simulink model "SensorFusion_Controller_Model"  (R2025a)
settings: Solver=VariableStepAuto  StartTime=0.0  StopTime=inf  FixedStep=1  RelTol=1e-3
undefined symbols (not defined in the file): DiscIntNeverNeededParam
libraries: simulink x17
(part 3 of 4)

== matlab function SensorFusion_Controller_Model/Sensor Fusion/Radar Sensor 1 ==
  data: dist input; elevation_live output; secondsCounter input; dayCounter input; water_lvl_live output; elevation_daily output
function [elevation_live, water_lvl_live, elevation_daily] = riverElevationSensor(dist, secondsCounter, dayCounter)

% INPUTS:
% dist - radar-measured distance from sensor to water surface (m) comes from the dashboard slider input
% secondsCounter - current second within the day (0 to 86399), from timer
% dayCounter- how many full days have passed, from timer
%
% OUTPUTS (LIVE that updates every timestep, use these for dashboard):
% elevation_live - current smoothed river water elevation in metres
% water_lvl_live - current water level status string (live, for dashboard)
%
% OUTPUTS (DAILY AVERAGE - updates once per day rollover, use for logger):
% elevation_daily - average river elevation across the entire previous day (m) computed as running sum 
% over 86400 seconds
%
% HOW IT WORKS:
% the sensor converts radar distance to river elevation using a fixed reference elevation (ref_elev).
% a smoothing factor gradually moves the elevation toward the target rather than jumping instantly,
% simulating real sensor lag. Every 86400 seconds (1 day), the current live values are saved as
% the daily snapshot before the timer resets.

ref_elev = 5.0; % height of sensor mount above riverbed (metres)
% water elevation = ref_elev - dist
MIN_ELEV = 0.0; % river physically cannot be below 0m
MAX_ELEV = 4.0; % maximum valid river level as defined by project spec

persistent prevSec prevDay elevation elevation_daily_store daily_sum daily_count

% initialise persistent variables
if isempty(prevSec), prevSec = 0; end
if isempty(prevDay), prevDay = 0; end
if isempty(elevation), elevation = ref_elev - dist; end
if isempty(elevation_daily_store), elevation_daily_store = 0; end
if isempty(daily_sum), daily_sum = 0; end
if isempty(daily_count), daily_count = 0; end

% time delta calculation
deltaT = secondsCounter - prevSec;
if deltaT <= 0
    deltaT = 1; % guard against zero or negative delta on reset tick
end

% target_elev is where the reading should be based on current dist input
target_elev = ref_elev - dist;

% clamp the target to valid physical range to prevents the slider going out of range
target_elev = max(MIN_ELEV, min(MAX_ELEV, target_elev));

% gradually move elevation toward target (smoothing factor = 100)
% a higher denominator = slower/smoother response to input changes
rate = (target_elev - elevation) / 100;
elevation = elevation + rate * deltaT;
elevation = max(MIN_ELEV, min(MAX_ELEV, elevation));

% Water level classification (based on live elevation) Thresholds (metres):
% elevation > 2.05 = Normal
% 1.70 < elevation <= 2.05 = Alert
% elevation <= 1.70 = Critical
if elevation > 2.05
    water_lvl_str = "Normal";
elseif elevation > 1.70
    water_lvl_str = "Alert";
else
    water_lvl_str = "Critical";
end

% add current elevation to running sum for daily average calculation
% Simulink calls this function every timestep so daily_sum accumulates all readings across the day,
% daily_count tracks how many readings taken
daily_sum   = daily_sum + elevation;
daily_count = daily_count + 1;

% daily average when the day counter increments
% when dayCounter changes, it means 86400s have passed and the timer reset for new day
if double(dayCounter) ~= double(prevDay)
    if daily_count > 0
        elevation_daily_store = daily_sum / daily_count; % true daily average
    end
    daily_sum   = 0; % reset accumulator for new day
    daily_count = 0; % reset sample counter for new day
    prevDay = double(dayCounter);
end

% update state for next timestep
prevSec = secondsCounter;

% assign outputs
% live outputs to the dashboard signals
elevation_live = elevation;
water_lvl_live = water_lvl_str;

% daily average output to the dailyLogger block
elevation_daily = elevation_daily_store;

end

== matlab function SensorFusion_Controller_Model/Sensor Fusion/MATLAB Function5 ==
  data: r1 input; elevation_fused_live output; r2 input; r3 input; fault_flags output; elevation_fused_daily output; dayCounter input
function [elevation_fused_live, fault_flags, elevation_fused_daily] = fuseRiverElevationSensors(r1, r2, r3, dayCounter)

% INPUTS:
% r1, r2, r3 - live elevation outputs from the 3 river sensor chains (m)
% dayCounter - how many full days have passed, from timer
%
% OUTPUTS (LIVE - updates every timestep, use for dashboard):
% elevation_fused_live - single best-estimate river elevation in metres
% fault_flags - [f1 f2 f3] boolean array, 1 = that sensor is flagged faulty
%
% OUTPUTS (DAILY AVERAGE - updates once per day rollover, use for logger):
% elevation_fused_daily - average fused river elevation across the entire day (m)
% computed as running sum / sample count over 86400 seconds
%
% HOW IT WORKS:
% 1. compute the mean of all 3 sensor readings
% 2. flag any sensor that deviates more than tolerance % from the mean as faulty
% 3. use only the non-faulty sensors to compute the fused value:
% - 3 valid = median
% - 2 valid = mean of the two
% - 1 valid = use that sensor directly
% - 0 valid = fallback to mean of all 3
% 4. hard clamp the output to [MIN_ELEV, MAX_ELEV] regardless of result
% to ensure no out-of-range value ever leaves this block
% 5. accumulate fused live value into running sum every timestep
% on dayCounter increment, compute daily average and reset accumulators

MIN_ELEV = 0.0;
MAX_ELEV = 4.0;
REF_HEIGHT = 5.0;

% fault detection tolerance
tol = 0.05; % sensor flagged if it deviates >5% from mean

% persistent variables for daily average tracking
persistent prevDay daily_sum daily_count fused_daily_store

% initialise persistent variables
if isempty(prevDay),          prevDay = 0;           end
if isempty(daily_sum),        daily_sum = 0;         end
if isempty(daily_count),      daily_count = 0;       end
if isempty(fused_daily_store),fused_daily_store = 0; end

% collect readings and calculate mean
vals = [r1, r2, r3];
mean_val = mean(vals);

% fault detection via comparing to tol % mean value
% use max(mean_val, 0.01) to avoid division by zero when mean is ~0
fault_flags = abs(vals - mean_val) > tol * max(mean_val, 0.01);

% fuse using only valid (non-faulty) sensors
valid_vals = vals(~fault_flags);
if isempty(valid_vals) % all 3 sensors flagged so fall back to best mean of all
    elevation_fused_live = mean_val;
elseif isscalar(valid_vals) % only 1 sensor valid, use it directly
    elevation_fused_live = valid_vals(1);
elseif numel(valid_vals) == 2 % 2 sensors valid, average them
    elevation_fused_live = mean(valid_vals);
else % all 3 sensors valid, use median
    elevation_fused_live = median(valid_vals);
end

% convert fused overhead distance to actual river level/depth
overhead_fused = elevation_fused_live;
elevation_fused_live = REF_HEIGHT - overhead_fused;

% output clamp
elevation_fused_live = max(MIN_ELEV, min(MAX_ELEV, elevation_fused_live));

% add fused value to running sum every timestep
% all readings across the day, daily_count tracks how many readings taken
daily_sum   = daily_sum + elevation_fused_live;
daily_count = daily_count + 1;

% daily average when dayCounter increments
if double(dayCounter) ~= double(prevDay)
    if daily_count > 0
        fused_daily_store = daily_sum / daily_count; % basically moving average
    end
    daily_sum   = 0; % reset accumulator for new day
    daily_count = 0; % reset sample counter for new day
    prevDay     = double(dayCounter);
end

% daily average output to dailyLogger block
elevation_fused_daily = fused_daily_store;

end

== matlab function SensorFusion_Controller_Model/Sensor Fusion/Soil Moisture Probe2 ==
  data: moisture_live output; moisture_type_live output; voltage_live output; sliderInput input; secondsCounter input; dayCounter input; moisture_daily output
function [moisture_live, moisture_type_live, voltage_live, moisture_daily] = soilMoistureProbe(sliderInput, ...
    secondsCounter, dayCounter)

% INPUTS:
% sliderInput - rainfall rate in mm/s from the dashboard slider
% secondsCounter - current second within the day (0 to 86399), from timer
% dayCounter - how many full days have passed, from timer
%
% OUTPUTS (LIVE which updates every timestep, use for dashboard):
% moisture_live - current soil moisture percentage (0 to 100%)
% moisture_type_live - current moisture category string (live)
% voltage_live - current sensor voltage output (live)
%
% OUTPUTS (DAILY - updates once per day rollover, use for logger):
% moisture_daily - end of day soil moisture % captured from previous tick
% scaled so max slider input (0.0012 mm/s) = 100% rounded to nearest whole 
% percentage
%
% HOW IT WORKS:
% Rainfall infiltrates into soil at a given efficiency rate, increasing the volumetric water content (VWC). 
% Evapotranspiration (ET) constantly draws moisture out. The resulting VWC is clamped to 0-100% and mapped
% to a moisture category and analog voltage every 86400 seconds the end-of-day values are snapshotted for 
% the logger
% on dayCounter increment, the daily value is captured from prev_moisture (previous tick's value)
% before resetting VWC to 0 for the new day, same pattern as tipping bucket.
% gain of 4.25 is applied so that max slider input (0.0012 mm/s) maps to 100%
% raw calculation gives 23.52% at max input, scale factor = 100/23.52 = 4.25

% constants
infil_eff = 0.7; % infiltration efficiency (70% of rain enters soil)
d = 300; % effective soil depth (mm)
ET_day = 2; % evapotranspiration loss per day (mm/day)
ET_rate = ET_day / 86400; % ET converted to per-second rate (mm/s)
gain = 4.25; % scale factor so max slider input = 100% (100/23.52 = 4.25)

persistent VWC prevSec prevDay moisture_daily_store prev_moisture

% initialise values
if isempty(VWC), VWC = 0; end
if isempty(prevSec), prevSec = 0; end
if isempty(prevDay), prevDay = 0; end
if isempty(moisture_daily_store), moisture_daily_store = 0; end
if isempty(prev_moisture), prev_moisture = 0; end

% time delta
deltaT = secondsCounter - prevSec;
if deltaT <= 0
    deltaT = 1;
end

% calculate how much rain falls and infiltrates in this timestep
rain_mm  = sliderInput * deltaT; % total rainfall in this timestep (mm)
infil_mm = infil_eff * rain_mm; % portion that actually enters the soil
rain_frac = infil_mm / d; % expressed as fraction of total soil depth

% calculate evapotranspiration loss in this timestep
ET_mm = ET_rate * deltaT; % moisture lost to ET this timestep (mm)
ET_frac = ET_mm / d; % expressed as fraction of total soil depth

% update cumulative volumetric water content in fraction
VWC = VWC + rain_frac - ET_frac;

% convert to raw percentage first (unscaled) for VWC writeback
moisture_pct_raw = VWC * 100;

% apply gain so max slider input = 100%, round and clamp
moisture_pct = round(moisture_pct_raw * gain);
moisture_pct = max(0, min(100, moisture_pct));

% write back using raw unscaled value so VWC accumulates correctly
% do NOT use moisture_pct here as it includes gain which would shrink VWC
VWC = moisture_pct_raw / 100;
VWC = max(0, VWC); % ensure VWC never goes negative

% moisture category classification
% 0  to < 25  = Dry
% 25 to < 50  = Moderate
% 50 to < 75  = Wet
% 75 to 100   = Saturated
if moisture_pct < 25
    moisture_type = "Dry";
elseif moisture_pct < 50
    moisture_type = "Moderate";
elseif moisture_pct < 75
    moisture_type = "Wet";
else
    moisture_type = "Saturated";
end

% voltage output
% 0% moisture = 0.5V
% 100% moisture = 1.5V
voltage = 0.5 + (moisture_pct / 100);

% daily value when the day counter increments
% prev_moisture holds value from previous tick before reset fires
% so we capture true end-of-day value, not post-reset zero
if double(dayCounter) ~= double(prevDay)
    moisture_daily_store = prev_moisture; % capture previous tick's value
    VWC = 0; % reset soil moisture for new day
    prevDay = double(dayCounter);
end

% update state for next timestep
prevSec = secondsCounter;
prev_moisture = moisture_pct; % store current value for next tick's capture

% assign outputs
% live outputs to the dashboard signals
moisture_live = moisture_pct;
moisture_type_live = moisture_type;
voltage_live = voltage;

% daily output to the dailyLogger block
moisture_daily = moisture_daily_store;

end

== matlab function SensorFusion_Controller_Model/Sensor Fusion/Tipping Bucket 1 ==
  data: sliderInput input; rainfall_live output; rainfall_daily output; secondsCounter input; dayCounter input; totalTipsDaily output
function [rainfall_live, rainfall_daily, totalTipsDaily] = tippingBucket1(sliderInput, secondsCounter, dayCounter)

% INPUTS:
% sliderInput - rainfall rate in mm/s from the dashboard slider
% secondsCounter - current second within the day (0 to 86399), from timer
% dayCounter - how many full days have passed, from timer
%
% OUTPUTS (LIVE - updates every timestep, use for dashboard):
% rainfall_live - running rainfall total today in mm
%
% OUTPUTS (DAILY TOTAL - updates once per day rollover, use for logger):
% rainfall_daily - total rainfall for the completed previous day (mm)
% totalTipsDaily  - total tips recorded for the completed previous day
%
% HOW IT WORKS:
% Rain accumulates in a virtual 0.2mm/tip bucket. Every time accumulated water reaches 0.2mm the bucket
% tips, incrementing the tip counter and subtracting 0.2mm from the accumulator.
% Total rainfall = tips * 0.2mm.
% On dayCounter increment, the daily total is captured from the PREVIOUS tick's value
% via prev_rainfall and prev_tips, before resetting counters for the new day.

TIP_VOL = 0.2; % each tip represents 0.2mm of rainfall

persistent acc tips prevSec prevDay rainfall_daily_store totalTips_store prev_rainfall prev_tips

if isempty(acc), acc = 0; end
if isempty(tips), tips = 0; end
if isempty(prevSec), prevSec = 0; end
if isempty(prevDay), prevDay = 0; end
if isempty(rainfall_daily_store), rainfall_daily_store = 0; end
if isempty(totalTips_store), totalTips_store = 0; end
if isempty(prev_rainfall), prev_rainfall = 0; end
if isempty(prev_tips), prev_tips = 0; end

deltaT = secondsCounter - prevSec;
if deltaT <= 0
    deltaT = 1; % guard against zero or negative delta on reset tick
end

% accumulate rainfall and count tips
acc = acc + sliderInput * deltaT;
while acc >= TIP_VOL
    tips = tips + 1; % one tip recorded
    acc  = acc - TIP_VOL; % remove one tip's worth from accumulator
end

% daily rollover to capture total then reset all counters for new day
if double(dayCounter) ~= double(prevDay)
    rainfall_daily_store = prev_rainfall; % capture today's total
    totalTips_store = prev_tips; % capture today's total tip count
    tips = 0; % reset tip counter for new day
    acc = 0; % reset accumulator for new day
    prevDay = double(dayCounter);
end

% update state for next timestep
prevSec = secondsCounter;
prev_rainfall = tips * TIP_VOL; % store current value for next tick's capture
prev_tips = tips; % store current tips for next tick's capture

% assign outputs
rainfall_live  = tips * TIP_VOL; % live running total for dashboard
rainfall_daily = rainfall_daily_store; % daily total for logger
totalTipsDaily = totalTips_store; % daily total tips for display

end

== matlab function SensorFusion_Controller_Model/Sensor Fusion/MATLAB Function6 ==
  data: noisy_input input; x_est output
function x_est = kalmanFilter(noisy_input)

persistent x P
if isempty(x), x = noisy_input; end
if isempty(P), P = 1; end


Q = 1e-10;   % process noise covariance
R = 1e-9;   % measurement noise covariance
% filter will trust measurement more since Q > R

% prediction
x_pred = x;
P_pred = P + Q;

% update
K = P_pred / (P_pred + R);
x = x_pred + K*(noisy_input - x_pred);
P = (1 - K)*P_pred;

x_est = max(0, x);

== matlab function SensorFusion_Controller_Model/Sensor Fusion/MATLAB Function7 ==
  data: noisy_input input; x_est output
function x_est = kalmanFilter(noisy_input)

persistent x P
if isempty(x), x = noisy_input; end
if isempty(P), P = 1; end


Q = 1e-10;   % process noise covariance
R = 1e-9;   % measurement noise covariance
% filter will trust measurement more since Q > R

% prediction
x_pred = x;
P_pred = P + Q;

% update
K = P_pred / (P_pred + R);
x = x_pred + K*(noisy_input - x_pred);
P = (1 - K)*P_pred;

x_est = max(0, x);

== matlab function SensorFusion_Controller_Model/Sensor Fusion/MATLAB Function8 ==
  data: r1 input; rainfall_fused_live output; r2 input; r3 input; fault_flags output; rainfall_fused_daily output; dayCounter input
function [rainfall_fused_live, fault_flags, rainfall_fused_daily] = fuseTippingBucketSensors(r1, r2, r3, dayCounter)
% INPUTS:
% r1, r2, r3 - rainfall_live outputs from the 3 tipping bucket chains (mm)
% dayCounter - how many full days have passed, from timer
%
% OUTPUTS (LIVE - updates every timestep, use for dashboard):
% rainfall_fused_live - single best-estimate running rainfall total in mm
% fault_flags - [f1 f2 f3] boolean array, 1 = that sensor is flagged faulty
%
% OUTPUTS (DAILY TOTAL - updates once per day rollover, use for logger):
% rainfall_fused_daily - total fused rainfall for the completed day (mm)
% captured from the previous tick before tippingBucket resets to 0
%
% HOW IT WORKS:
% same structure as the other fusion blocks with 10% tolerance only unlike soil moisture and river
% elevation and the daily value is a total
% prev_fused stores the fused value from the previous tick so that when
% dayCounter increments on the same tick that sensors reset to 0, we
% capture the true end-of-day total rather than the post-reset zero

% limits
MIN_RAIN = 0.0;
MAX_RAIN = Inf;

% fault detection tolerance
tol = 0.10;
abs_floor = 0.4; % 0.4mm absolute floor to prevents false fault at near-zero

% persistent variables for daily total tracking
persistent prevDay fused_daily_store prev_fused

% initialise persistent variables
if isempty(prevDay), prevDay = 0; end
if isempty(fused_daily_store), fused_daily_store = 0; end
if isempty(prev_fused), prev_fused = 0; end

% calculate mean
vals = [r1, r2, r3];
mean_val = mean(vals);

% fault detection
% sensor is faulty if BOTH the relative AND absolute deviations are large
% using AND logic prevents flagging sensors just because of tiny 0.2mm tip
% differences when all sensors are essentially reading the same thing
rel_dev = abs(vals - mean_val) > tol * max(mean_val, 0.01);
abs_dev = abs(vals - mean_val) > abs_floor;
fault_flags = rel_dev & abs_dev;

% fuse using only valid sensors
valid_vals = vals(~fault_flags);
if isempty(valid_vals)
    rainfall_fused_live = mean_val;
elseif isscalar(valid_vals)
    rainfall_fused_live = valid_vals(1);
elseif numel(valid_vals) == 2
    rainfall_fused_live = mean(valid_vals);
else
    rainfall_fused_live = median(valid_vals);
end

% output clamp
rainfall_fused_live = max(MIN_RAIN, rainfall_fused_live);

% daily total when dayCounter increments
% prev_fused holds the fused value from the tick before the reset
% so we capture the true end-of-day total, not the post-reset 0
if double(dayCounter) ~= double(prevDay)
    fused_daily_store = prev_fused; % use previous tick's value
    prevDay = double(dayCounter);
end

% store current fused value for next tick's capture
prev_fused = rainfall_fused_live;

% daily total output to dailyLogger block
rainfall_fused_daily = fused_daily_store;

end

== matlab function SensorFusion_Controller_Model/Sensor Fusion/Soil Moisture Probe3 ==
  data: moisture_live output; moisture_type_live output; voltage_live output; sliderInput input; secondsCounter input; dayCounter input; moisture_daily output
function [moisture_live, moisture_type_live, voltage_live, moisture_daily] = soilMoistureProbe(sliderInput, ...
    secondsCounter, dayCounter)

% INPUTS:
% sliderInput - rainfall rate in mm/s from the dashboard slider
% secondsCounter - current second within the day (0 to 86399), from timer
% dayCounter - how many full days have passed, from timer
%
% OUTPUTS (LIVE which updates every timestep, use for dashboard):
% moisture_live - current soil moisture percentage (0 to 100%)
% moisture_type_live - current moisture category string (live)
% voltage_live - current sensor voltage output (live)
%
% OUTPUTS (DAILY - updates once per day rollover, use for logger):
% moisture_daily - end of day soil moisture % captured from previous tick
% scaled so max slider input (0.0012 mm/s) = 100% rounded to nearest whole 
% percentage
%
% HOW IT WORKS:
% Rainfall infiltrates into soil at a given efficiency rate, increasing the volumetric water content (VWC). 
% Evapotranspiration (ET) constantly draws moisture out. The resulting VWC is clamped to 0-100% and mapped
% to a moisture category and analog voltage every 86400 seconds the end-of-day values are snapshotted for 
% the logger
% on dayCounter increment, the daily value is captured from prev_moisture (previous tick's value)
% before resetting VWC to 0 for the new day, same pattern as tipping bucket.
% gain of 4.25 is applied so that max slider input (0.0012 mm/s) maps to 100%
% raw calculation gives 23.52% at max input, scale factor = 100/23.52 = 4.25

% constants
infil_eff = 0.7; % infiltration efficiency (70% of rain enters soil)
d = 300; % effective soil depth (mm)
ET_day = 2; % evapotranspiration loss per day (mm/day)
ET_rate = ET_day / 86400; % ET converted to per-second rate (mm/s)
gain = 4.25; % scale factor so max slider input = 100% (100/23.52 = 4.25)

persistent VWC prevSec prevDay moisture_daily_store prev_moisture

% initialise values
if isempty(VWC), VWC = 0; end
if isempty(prevSec), prevSec = 0; end
if isempty(prevDay), prevDay = 0; end
if isempty(moisture_daily_store), moisture_daily_store = 0; end
if isempty(prev_moisture), prev_moisture = 0; end

% time delta
deltaT = secondsCounter - prevSec;
if deltaT <= 0
    deltaT = 1;
end

% calculate how much rain falls and infiltrates in this timestep
rain_mm  = sliderInput * deltaT; % total rainfall in this timestep (mm)
infil_mm = infil_eff * rain_mm; % portion that actually enters the soil
rain_frac = infil_mm / d; % expressed as fraction of total soil depth

% calculate evapotranspiration loss in this timestep
ET_mm = ET_rate * deltaT; % moisture lost to ET this timestep (mm)
ET_frac = ET_mm / d; % expressed as fraction of total soil depth

% update cumulative volumetric water content in fraction
VWC = VWC + rain_frac - ET_frac;

% convert to raw percentage first (unscaled) for VWC writeback
moisture_pct_raw = VWC * 100;

% apply gain so max slider input = 100%, round and clamp
moisture_pct = round(moisture_pct_raw * gain);
moisture_pct = max(0, min(100, moisture_pct));

% write back using raw unscaled value so VWC accumulates correctly
% do NOT use moisture_pct here as it includes gain which would shrink VWC
VWC = moisture_pct_raw / 100;
VWC = max(0, VWC); % ensure VWC never goes negative

% moisture category classification
% 0  to < 25  = Dry
% 25 to < 50  = Moderate
% 50 to < 75  = Wet
% 75 to 100   = Saturated
if moisture_pct < 25
    moisture_type = "Dry";
elseif moisture_pct < 50
    moisture_type = "Moderate";
elseif moisture_pct < 75
    moisture_type = "Wet";
else
    moisture_type = "Saturated";
end

% voltage output
% 0% moisture = 0.5V
% 100% moisture = 1.5V
voltage = 0.5 + (moisture_pct / 100);

% daily value when the day counter increments
% prev_moisture holds value from previous tick before reset fires
% so we capture true end-of-day value, not post-reset zero
if double(dayCounter) ~= double(prevDay)
    moisture_daily_store = prev_moisture; % capture previous tick's value
    VWC = 0; % reset soil moisture for new day
    prevDay = double(dayCounter);
end

% update state for next timestep
prevSec = secondsCounter;
prev_moisture = moisture_pct; % store current value for next tick's capture

% assign outputs
% live outputs to the dashboard signals
moisture_live = moisture_pct;
moisture_type_live = moisture_type;
voltage_live = voltage;

% daily output to the dailyLogger block
moisture_daily = moisture_daily_store;

end

== matlab function SensorFusion_Controller_Model/Sensor Fusion/Soil Moisture Probe1 ==
  data: moisture_live output; moisture_type_live output; voltage_live output; sliderInput input; secondsCounter input; dayCounter input; moisture_daily output
function [moisture_live, moisture_type_live, voltage_live, moisture_daily] = soilMoistureProbe(sliderInput, ...
    secondsCounter, dayCounter)

% INPUTS:
% sliderInput - rainfall rate in mm/s from the dashboard slider
% secondsCounter - current second within the day (0 to 86399), from timer
% dayCounter - how many full days have passed, from timer
%
% OUTPUTS (LIVE which updates every timestep, use for dashboard):
% moisture_live - current soil moisture percentage (0 to 100%)
% moisture_type_live - current moisture category string (live)
% voltage_live - current sensor voltage output (live)
%
% OUTPUTS (DAILY - updates once per day rollover, use for logger):
% moisture_daily - end of day soil moisture % captured from previous tick
% scaled so max slider input (0.0012 mm/s) = 100% rounded to nearest whole 
% percentage
%
% HOW IT WORKS:
% Rainfall infiltrates into soil at a given efficiency rate, increasing the volumetric water content (VWC). 
% Evapotranspiration (ET) constantly draws moisture out. The resulting VWC is clamped to 0-100% and mapped
% to a moisture category and analog voltage every 86400 seconds the end-of-day values are snapshotted for 
% the logger
% on dayCounter increment, the daily value is captured from prev_moisture (previous tick's value)
% before resetting VWC to 0 for the new day, same pattern as tipping bucket.
% gain of 4.25 is applied so that max slider input (0.0012 mm/s) maps to 100%
% raw calculation gives 23.52% at max input, scale factor = 100/23.52 = 4.25

% constants
infil_eff = 0.7; % infiltration efficiency (70% of rain enters soil)
d = 300; % effective soil depth (mm)
ET_day = 2; % evapotranspiration loss per day (mm/day)
ET_rate = ET_day / 86400; % ET converted to per-second rate (mm/s)
gain = 4.25; % scale factor so max slider input = 100% (100/23.52 = 4.25)

persistent VWC prevSec prevDay moisture_daily_store prev_moisture

% initialise values
if isempty(VWC), VWC = 0; end
if isempty(prevSec), prevSec = 0; end
if isempty(prevDay), prevDay = 0; end
if isempty(moisture_daily_store), moisture_daily_store = 0; end
if isempty(prev_moisture), prev_moisture = 0; end

% time delta
deltaT = secondsCounter - prevSec;
if deltaT <= 0
    deltaT = 1;
end

% calculate how much rain falls and infiltrates in this timestep
rain_mm  = sliderInput * deltaT; % total rainfall in this timestep (mm)
infil_mm = infil_eff * rain_mm; % portion that actually enters the soil
rain_frac = infil_mm / d; % expressed as fraction of total soil depth

% calculate evapotranspiration loss in this timestep
ET_mm = ET_rate * deltaT; % moisture lost to ET this timestep (mm)
ET_frac = ET_mm / d; % expressed as fraction of total soil depth

% update cumulative volumetric water content in fraction
VWC = VWC + rain_frac - ET_frac;

% convert to raw percentage first (unscaled) for VWC writeback
moisture_pct_raw = VWC * 100;

% apply gain so max slider input = 100%, round and clamp
moisture_pct = round(moisture_pct_raw * gain);
moisture_pct = max(0, min(100, moisture_pct));

% write back using raw unscaled value so VWC accumulates correctly
% do NOT use moisture_pct here as it includes gain which would shrink VWC
VWC = moisture_pct_raw / 100;
VWC = max(0, VWC); % ensure VWC never goes negative

% moisture category classification
% 0  to < 25  = Dry
% 25 to < 50  = Moderate
% 50 to < 75  = Wet
% 75 to 100   = Saturated
if moisture_pct < 25
    moisture_type = "Dry";
elseif moisture_pct < 50
    moisture_type = "Moderate";
elseif moisture_pct < 75
    moisture_type = "Wet";
else
    moisture_type = "Saturated";
end

% voltage output
% 0% moisture = 0.5V
% 100% moisture = 1.5V
voltage = 0.5 + (moisture_pct / 100);

% daily value when the day counter increments
% prev_moisture holds value from previous tick before reset fires
% so we capture true end-of-day value, not post-reset zero
if double(dayCounter) ~= double(prevDay)
    moisture_daily_store = prev_moisture; % capture previous tick's value
    VWC = 0; % reset soil moisture for new day
    prevDay = double(dayCounter);
end

% update state for next timestep
prevSec = secondsCounter;
prev_moisture = moisture_pct; % store current value for next tick's capture

% assign outputs
% live outputs to the dashboard signals
moisture_live = moisture_pct;
moisture_type_live = moisture_type;
voltage_live = voltage;

% daily output to the dailyLogger block
moisture_daily = moisture_daily_store;

end

== matlab function SensorFusion_Controller_Model/Sensor Fusion/MATLAB Function9 ==
  data: noisy_input input; x_est output
function x_est = kalmanFilter(noisy_input)

persistent x P
if isempty(x), x = noisy_input; end
if isempty(P), P = 1; end


Q = 1e-10;   % process noise covariance
R = 1e-9;   % measurement noise covariance
% filter will trust measurement more since Q > R

% prediction
x_pred = x;
P_pred = P + Q;

% update
K = P_pred / (P_pred + R);
x = x_pred + K*(noisy_input - x_pred);
P = (1 - K)*P_pred;

x_est = max(0, x);

== matlab function SensorFusion_Controller_Model/Sensor Fusion/MATLAB Function10 ==
  data: noisy_input input; x_est output
function x_est = kalmanFilter(noisy_input)

persistent x P
if isempty(x), x = noisy_input; end
if isempty(P), P = 1; end


Q = 1e-10;   % process noise covariance
R = 1e-9;   % measurement noise covariance
% filter will trust measurement more since Q > R

% prediction
x_pred = x;
P_pred = P + Q;

% update
K = P_pred / (P_pred + R);
x = x_pred + K*(noisy_input - x_pred);
P = (1 - K)*P_pred;

x_est = max(0, x);

== matlab function SensorFusion_Controller_Model/Sensor Fusion/Daily Logger ==
  data: rv1_daily input; rv2_daily input; rv3_daily input; tb1_daily input; tb2_daily input; tb3_daily input; sm1_daily input; sm2_daily input; sm3_daily input; rv_fused_daily input; tb_fused_daily input; sm_fused_daily input; dayCounter input
function dailyLogger(rv1_daily, rv2_daily, rv3_daily, tb1_daily, tb2_daily, tb3_daily, sm1_daily, sm2_daily, sm3_daily, ...
    rv_fused_daily, tb_fused_daily, sm_fused_daily, dayCounter)

% INPUTS:
% dayCounter - how many full days have passed (from timer block)
%
% tb1_daily, tb2_daily, tb3_daily - rainfall_daily from each of the 3 tipping bucket sensors (mm)
% total rainfall accumulated over the entire day
%
% sm1_daily, sm2_daily, sm3_daily - moisture_daily from each of the 3 soil moisture sensors (%)
% average soil moisture % across the entire day
%
% rv1_daily, rv2_daily, rv3_daily - elevation_daily from each of the 3 river elevation sensors (m)
% average river elevation across the entire day
%
% tb_fused_daily - fused tipping bucket daily total (mm) captured at day rollover from 
% fuseTippingBucketSensors
%
% sm_fused_daily - fused soil moisture daily average (%) computed as running sum in 
% fuseSoilMoistSensors
%
% rv_fused_daily - fused river elevation daily average (m) computed as running sum in 
% fuseRiverElevationSensors
%
% OUTPUT:
% writes one row per day to flood_sensor_log.csv in the MATLAB working directory. the file is 
% created from day 1 and appended every day after that. open the CSV directly in Excel or 
% import into any tool.
%
% HOW IT WORKS:
% this function is called every timestep but only acts when the reset signal goes high (reset == 1)
% AND the day number has changed. The persistent lastDay ensures it fires exactly once per day,
% even if the reset signal stays high for multiple ticks

% allow MATLAB-only functions during simulation (fix for Simulink codegen)
coder.extrinsic('datetime','datestr','fopen','fprintf','fclose','warning');

% log file configuration
filename = 'flood_sensor_log.csv';

% persistent to prevent duplicate writes within one reset tick
persistent lastDay
if isempty(lastDay)
    lastDay = -1; % use -1 so it does not skip day 0
end

% only proceed when dayCounter increments (new day detected)
if double(dayCounter) == lastDay || double(dayCounter) == 0 % additional guard to not skip day 0
    return; % do nothing since same as last day
end

% mark this day as logged so we dont write again until next day
lastDay = double(dayCounter);

% build timestamp string for this log entry
% uses real wall-clock time so entries can be correlated to actual test or deployment time, not 
% just simulation time
timestamp = char(zeros(1,19));

t = datetime('now');
timestamp = datestr(t, 'yyyy-mm-dd HH:MM:SS');

% write header row on the very first day only
if double(dayCounter) == 1

    fid = -1;
    fid = fopen(filename, 'w'); % 'w' = create new / overwrite

    if fid ~= -1
        fprintf(fid, [ ...
            'Timestamp,'        ...
            'Day,'              ...
            'TB1_mm,'           ...    % Tipping Bucket sensor 1 - total daily rainfall (mm)
            'TB2_mm,'           ...    % Tipping Bucket sensor 2 - total daily rainfall (mm)
            'TB3_mm,'           ...    % Tipping Bucket sensor 3 - total daily rainfall (mm)
            'TB_Fused_mm,'      ...    % Fused tipping bucket - total daily rainfall (mm)
            'SM1_pct,'          ...    % Soil Moisture sensor 1 - average daily moisture (%)
            'SM2_pct,'          ...    % Soil Moisture sensor 2 - average daily moisture (%)
            'SM3_pct,'          ...    % Soil Moisture sensor 3 - average daily moisture (%)
            'SM_Fused_pct,'     ...    % Fused soil moisture - average daily moisture (%)
            'RV1_m,'            ...    % River Elevation sensor 1 - average daily elevation (m)
            'RV2_m,'            ...    % River Elevation sensor 2 - average daily elevation (m)
            'RV3_m,'            ...    % River Elevation sensor 3 - average daily elevation (m)
            'RV_Fused_m\n'      ...    % Fused river elevation - average daily elevation (m)
        ]);
        fclose(fid);
    else
        warning('dailyLogger: Could not open file for writing.');
    end

end

% append the data row for this day
fid = -1;
fid = fopen(filename, 'a'); % 'a' = append so it never overwrites existing rows

if fid ~= -1
    fprintf(fid, '%s,%d,%.4f,%.4f,%.4f,%.4f,%.4f,%.4f,%.4f,%.4f,%.4f,%.4f,%.4f,%.4f\n', ...
        timestamp,          ...     % wall-clock time of this log entry
        double(dayCounter), ...     % simulation day number
        tb1_daily,          ...     % tipping bucket sensor 1 total (mm)
        tb2_daily,          ...     % tipping bucket sensor 2 total (mm)
        tb3_daily,          ...     % tipping bucket sensor 3 total (mm)
        tb_fused_daily,     ...     % fused tipping bucket total (mm)
        sm1_daily,          ...     % soil moisture sensor 1 average (%)
        sm2_daily,          ...     % soil moisture sensor 2 average (%)
        sm3_daily,          ...     % soil moisture sensor 3 average (%)
        sm_fused_daily,     ...     % fused soil moisture average (%)
        rv1_daily,          ...     % river elevation sensor 1 average (m)
        rv2_daily,          ...     % river elevation sensor 2 average (m)
        rv3_daily,          ...     % river elevation sensor 3 average (m)
        rv_fused_daily      ...     % fused river elevation average (m)
    );

    fclose(fid);
else
    warning('dailyLogger: Could not open file for appending.');
end

% console confirmation so can verify logging is working during testing
% remove or comment this line out once confirmed working in production
fprintf('[dailyLogger] Day %d logged at %s\n', double(dayCounter), timestamp);

end

== matlab function SensorFusion_Controller_Model/Sensor Fusion/MATLAB Function12 ==
  data: r1 input; moisture_fused_live output; r2 input; r3 input; fault_flags output; moisture_fused_daily output; dayCounter input
function [moisture_fused_live, fault_flags, moisture_fused_daily] = fuseSoilMoistSensors(r1, r2, r3, dayCounter)

% INPUTS:
% r1, r2, r3 - live moisture_live outputs from the 3 soil sensor chains (%)
% dayCounter - how many full days have passed, from timer
%
% OUTPUTS (LIVE - updates every timestep, use for dashboard):
% moisture_fused_live - single best-estimate soil moisture percentage (0-100%)
% fault_flags - [f1 f2 f3] boolean array, 1 = that sensor is flagged faulty
%
% OUTPUTS (DAILY - updates once per day rollover, use for logger):
% moisture_fused_daily - fused soil moisture % captured from previous tick before reset
% consistent with tipping bucket approach using prev_fused
%
% HOW IT WORKS:
% same fault-detection and fusion logic as fuseRiverElevationSensors, but with a wider 13% tolerance because
% soil moisture varies more naturally across sensor placement locations
% output is clamped to 0-100% to not exceed bounds
% prev_fused holds the fused value from the previous tick so when dayCounter
% increments on the same tick that sensors reset to 0, we capture the true
% end-of-day value rather than the post-reset zero

% limits
MIN_MOIST = 0.0;
MAX_MOIST = 100.0;

% fault detection tolerance
tol = 0.13;

% persistent variables for daily tracking
persistent prevDay fused_daily_store prev_fused

% initialise persistent variables
if isempty(prevDay), prevDay = 0; end
if isempty(fused_daily_store), fused_daily_store = 0; end
if isempty(prev_fused), prev_fused = 0; end

% find mean
vals = [r1, r2, r3];
mean_val = mean(vals);

% fault detection
fault_flags = abs(vals - mean_val) > tol * max(mean_val, 0.01);

% fuse using only valid sensors
valid_vals = vals(~fault_flags);
if isempty(valid_vals)
    moisture_fused_live = mean_val;
elseif isscalar(valid_vals)
    moisture_fused_live = valid_vals(1);
elseif numel(valid_vals) == 2
    moisture_fused_live = mean(valid_vals);
else
    moisture_fused_live = median(valid_vals);
end

% output clamp
moisture_fused_live = max(MIN_MOIST, min(MAX_MOIST, moisture_fused_live));

% daily value when dayCounter increments
% prev_fused holds the fused value from the tick before the reset
% so we capture the true end-of-day value, not the post-reset 0
if double(dayCounter) ~= double(prevDay)
    fused_daily_store = prev_fused; % use previous tick's value
    prevDay = double(dayCounter);
end

% store current fused value for next tick's capture
prev_fused = moisture_fused_live;

% daily output to dailyLogger block
moisture_fused_daily = fused_daily_store;

end

== matlab function SensorFusion_Controller_Model/Sensor Fusion/Tipping Bucket 2 ==
  data: sliderInput input; rainfall_live output; rainfall_daily output; secondsCounter input; dayCounter input; totalTipsDaily output
function [rainfall_live, rainfall_daily, totalTipsDaily] = tippingBucket1(sliderInput, secondsCounter, dayCounter)

% INPUTS:
% sliderInput - rainfall rate in mm/s from the dashboard slider
% secondsCounter - current second within the day (0 to 86399), from timer
% dayCounter - how many full days have passed, from timer
%
% OUTPUTS (LIVE - updates every timestep, use for dashboard):
% rainfall_live - running rainfall total today in mm
%
% OUTPUTS (DAILY TOTAL - updates once per day rollover, use for logger):
% rainfall_daily - total rainfall for the completed previous day (mm)
% totalTipsDaily  - total tips recorded for the completed previous day
%
% HOW IT WORKS:
% Rain accumulates in a virtual 0.2mm/tip bucket. Every time accumulated water reaches 0.2mm the bucket
% tips, incrementing the tip counter and subtracting 0.2mm from the accumulator.
% Total rainfall = tips * 0.2mm.
% On dayCounter increment, the daily total is captured from the PREVIOUS tick's value
% via prev_rainfall and prev_tips, before resetting counters for the new day.

TIP_VOL = 0.2; % each tip represents 0.2mm of rainfall

persistent acc tips prevSec prevDay rainfall_daily_store totalTips_store prev_rainfall prev_tips

if isempty(acc), acc = 0; end
if isempty(tips), tips = 0; end
if isempty(prevSec), prevSec = 0; end
if isempty(prevDay), prevDay = 0; end
if isempty(rainfall_daily_store), rainfall_daily_store = 0; end
if isempty(totalTips_store), totalTips_store = 0; end
if isempty(prev_rainfall), prev_rainfall = 0; end
if isempty(prev_tips), prev_tips = 0; end

deltaT = secondsCounter - prevSec;
if deltaT <= 0
    deltaT = 1; % guard against zero or negative delta on reset tick
end

% accumulate rainfall and count tips
acc = acc + sliderInput * deltaT;
while acc >= TIP_VOL
    tips = tips + 1; % one tip recorded
    acc  = acc - TIP_VOL; % remove one tip's worth from accumulator
end

% daily rollover to capture total then reset all counters for new day
if double(dayCounter) ~= double(prevDay)
    rainfall_daily_store = prev_rainfall; % capture today's total
    totalTips_store = prev_tips; % capture today's total tip count
    tips = 0; % reset tip counter for new day
    acc = 0; % reset accumulator for new day
    prevDay = double(dayCounter);
end

% update state for next timestep
prevSec = secondsCounter;
prev_rainfall = tips * TIP_VOL; % store current value for next tick's capture
prev_tips = tips; % store current tips for next tick's capture

% assign outputs
rainfall_live  = tips * TIP_VOL; % live running total for dashboard
rainfall_daily = rainfall_daily_store; % daily total for logger
totalTipsDaily = totalTips_store; % daily total tips for display

end

== matlab function SensorFusion_Controller_Model/Sensor Fusion/MATLAB Function13 ==
  data: noisy_input input; x_est output
function x_est = kalmanFilter(noisy_input)

persistent x P
if isempty(x), x = noisy_input; end
if isempty(P), P = 1; end


Q = 1e-10;   % process noise covariance
R = 1e-9;   % measurement noise covariance
% filter will trust measurement more since Q > R

% prediction
x_pred = x;
P_pred = P + Q;

% update
K = P_pred / (P_pred + R);
x = x_pred + K*(noisy_input - x_pred);
P = (1 - K)*P_pred;

x_est = max(0, x);

== matlab function SensorFusion_Controller_Model/Sensor Fusion/Tipping Bucket 3 ==
  data: sliderInput input; rainfall_live output; rainfall_daily output; secondsCounter input; dayCounter input; totalTipsDaily output
function [rainfall_live, rainfall_daily, totalTipsDaily] = tippingBucket1(sliderInput, secondsCounter, dayCounter)

% INPUTS:
% sliderInput - rainfall rate in mm/s from the dashboard slider
% secondsCounter - current second within the day (0 to 86399), from timer
% dayCounter - how many full days have passed, from timer
%
% OUTPUTS (LIVE - updates every timestep, use for dashboard):
% rainfall_live - running rainfall total today in mm
%
% OUTPUTS (DAILY TOTAL - updates once per day rollover, use for logger):
% rainfall_daily - total rainfall for the completed previous day (mm)
% totalTipsDaily  - total tips recorded for the completed previous day
%
% HOW IT WORKS:
% Rain accumulates in a virtual 0.2mm/tip bucket. Every time accumulated water reaches 0.2mm the bucket
% tips, incrementing the tip counter and subtracting 0.2mm from the accumulator.
% Total rainfall = tips * 0.2mm.
% On dayCounter increment, the daily total is captured from the PREVIOUS tick's value
% via prev_rainfall and prev_tips, before resetting counters for the new day.

TIP_VOL = 0.2; % each tip represents 0.2mm of rainfall

persistent acc tips prevSec prevDay rainfall_daily_store totalTips_store prev_rainfall prev_tips

if isempty(acc), acc = 0; end
if isempty(tips), tips = 0; end
if isempty(prevSec), prevSec = 0; end
if isempty(prevDay), prevDay = 0; end
if isempty(rainfall_daily_store), rainfall_daily_store = 0; end
if isempty(totalTips_store), totalTips_store = 0; end
if isempty(prev_rainfall), prev_rainfall = 0; end
if isempty(prev_tips), prev_tips = 0; end

deltaT = secondsCounter - prevSec;
if deltaT <= 0
    deltaT = 1; % guard against zero or negative delta on reset tick
end

% accumulate rainfall and count tips
acc = acc + sliderInput * deltaT;
while acc >= TIP_VOL
    tips = tips + 1; % one tip recorded
    acc  = acc - TIP_VOL; % remove one tip's worth from accumulator
end

% daily rollover to capture total then reset all counters for new day
if double(dayCounter) ~= double(prevDay)
    rainfall_daily_store = prev_rainfall; % capture today's total
    totalTips_store = prev_tips; % capture today's total tip count
    tips = 0; % reset tip counter for new day
    acc = 0; % reset accumulator for new day
    prevDay = double(dayCounter);
end

% update state for next timestep
prevSec = secondsCounter;
prev_rainfall = tips * TIP_VOL; % store current value for next tick's capture
prev_tips = tips; % store current tips for next tick's capture

% assign outputs
rainfall_live  = tips * TIP_VOL; % live running total for dashboard
rainfall_daily = rainfall_daily_store; % daily total for logger
totalTipsDaily = totalTips_store; % daily total tips for display

end

== stateflow chart SensorFusion_Controller_Model/Rule Based Flood Controller_2/Water Pump and Sluice Gate Controller ==
  state AUTO_MODE
    entry:
    controlMode=0;
    state NORMAL
      entry:
      PumpCmd=0;
      GateCmd=0;
      Auto_SirenCmd=false;
    state AI_EARLY_MITIGATION
      entry:
      AI_EarlyMitigationActive=1;
      during:
      controlMode = 0;
      PumpCmd = 0;
      GateCmd = 0;
      Auto_SirenCmd = false;
      if Rainfall_Norm >= 0.8 && RiverLevel_Norm >= 0.8
      PumpCmd = 1;
      GateCmd = 1;
      elseif Rainfall_Norm >= RiverLevel_Norm
      PumpCmd = 1;
      else
      GateCmd = 1;
      end
      exit:
      AI_EarlyMitigationActive=0;
    state ALERT
      during:
      PumpCmd = 0;
      GateCmd = 0;
      Auto_SirenCmd = false;
      if Flood_Type == 1
      GateCmd = 1;      % 30%
      elseif Flood_Type == 2
      PumpCmd = 1;      % 30%
      elseif Flood_Type == 3
      PumpCmd = 1;      % 30%
      GateCmd = 1;      % 30%
      end
    state WARNING
      during:
      PumpCmd = 0;
      GateCmd = 0;
      Auto_SirenCmd = false;
      if Flood_Type == 1
      GateCmd = 2;      % 70%
      elseif Flood_Type == 2
      PumpCmd = 2;      % 70%
      elseif Flood_Type == 3
      PumpCmd = 2;      % 70%
      GateCmd = 2;      % 70%
      end
    state DANGER
      entry:
      PumpCmd = 3;          % 100%
      GateCmd = 3;          % 100%
      Auto_SirenCmd = true;
    (default) -> NORMAL
    AI_EARLY_MITIGATION -> NORMAL [order 1] : [AI_FloodFlag == 0 || Confidence <= 0.3]
    NORMAL -> AI_EARLY_MITIGATION [order 2] : [FRI < 0.3 && AI_FloodFlag==1&&Confidence>0.61]
    ALERT -> NORMAL [order 2] : [FRI < 0.29]
    NORMAL -> ALERT [order 1] : [FRI >= 0.3]
    AI_EARLY_MITIGATION -> ALERT [order 2] : [FRI >= 0.3]
    WARNING -> ALERT [order 2] : [FRI < 0.56]
    ALERT -> WARNING [order 1] : [FRI >= 0.6]
    DANGER -> WARNING : [FRI <= 0.76]
    WARNING -> DANGER [order 1] : [FRI >= 0.8]
  state MANUAL_MODE
    state MANUAL_MODE
      during:
      controlMode = 1;
      PumpCmd = Manual_PumpLevel;
      GateCmd = Manual_GateLevel;
      if Manual_PumpLevel > 3
      PumpCmd = 0;
      else
      PumpCmd = Manual_PumpLevel;
      end
      if Manual_GateLevel > 3
      GateCmd = 0;
      else
      GateCmd = Manual_GateLevel;
      end
    (default) -> MANUAL_MODE.MANUAL_MODE
  (default) -> AUTO_MODE
  AUTO_MODE -> MANUAL_MODE : [Manual_Enable==1]
  MANUAL_MODE -> AUTO_MODE : [Manual_Enable==0]
  data: FRI input; Flood_Type input; PumpCmd output; GateCmd output; Auto_SirenCmd output; Manual_Enable input; controlMode output; Manual_GateLevel input; Manual_PumpLevel input; AI_FloodFlag input; Confidence input; AI_EarlyMitigationActive output; Rainfall_Norm input; RiverLevel_Norm input

== matlab function SensorFusion_Controller_Model/Sensor Fusion/MATLAB Function1 ==
  data: noisy_input input; x_est output
function x_est = kalmanFilter(noisy_input)

persistent x P
if isempty(x), x = noisy_input; end
if isempty(P), P = 1; end


Q = 1e-10;   % process noise covariance
R = 1e-9;   % measurement noise covariance
% filter will trust measurement more since Q > R

% prediction
x_pred = x;
P_pred = P + Q;

% update
K = P_pred / (P_pred + R);
x = x_pred + K*(noisy_input - x_pred);
P = (1 - K)*P_pred;

x_est = max(0, x);
